simulink model "QPSK_delayChannel"  (R2017b)
settings: Solver=FixedStepDiscrete  StartTime=0.0  StopTime=inf  RelTol=1e-3
PreLoadFcn:
  | sdrqpsktx = sdrzqpsktxFMC234_init;
  | sdrqpskrx = sdrzqpskrxFMC234_init;
InitFcn:
  | sdrqpsktx = sdrzqpsktxFMC234_init;
  | sdrqpskrx = sdrzqpskrxFMC234_init;
undefined symbols (not defined in the file or in its folder): dfilt, gcbh, rcfiltgaincompat
libraries: commdigbbndpm3 x3, dspstat3 x3, dspobslib x3, dspsigops x2, commsequence2 x2, commutil2 x2, commfilt2 x2, simulink x2, commrfcorlib x1, commrflib2 x1, commblksprivate x1, dspspect3 x1
Description:
  | Implement a QPSK Transmitter prototype using SDR hardware
settings Model: FPTRunName=Active  ModifiedByFormat=The MathWorks Inc.  SimulationMode=accelerator  Creator=The MathWorks, Inc.  LastModifiedBy=The MathWorks Inc.
settings DataIOCC: LimitDataPoints=on  SaveFormat=Array  SaveOutput=off  SaveTime=off
settings OptimizationCC: BooleanDataType=off  DefaultParameterBehavior=Inlined  ExpressionDepthLimit=2147483647  LocalBlockOutputs=off  LifeSpan=inf
settings DebuggingCC: AlgebraicLoopMsg=error  UnderspecifiedInitializationDetection=Classic  MergeDetectMultiDrivingBlocksExec=none  SolverPrmCheckMsg=warning  SingleTaskRateTransMsg=error  FcnCallInpInsideContextMsg=warning  AllowSymbolicDim=off  StateNameClashWarn=warning  SFUnexpectedBacktrackingDiag=warning  SFNoUnconditionalDefaultTransitionDiag=warning  SFExecutionAtInitializationDiag=none
settings HardwareCC: ProdBitPerPointer=32  ProdBitPerSizeT=32  ProdBitPerPtrDiffT=32  ProdLargestAtomicFloat=None  ProdIntDivRoundTo=Undefined  ProdEndianess=Unspecified  ProdWordSize=32  ProdHWDeviceType=32-bit Generic  TargetBitPerPointer=64  TargetBitPerSizeT=64  TargetBitPerPtrDiffT=64  TargetLongLongMode=on  TargetIntDivRoundTo=Zero  TargetEndianess=LittleEndian  TargetWordSize=64  TargetHWDeviceType=Generic->MATLAB Host Computer  ProdEqTarget=off
settings ModelReferenceCC: PropagateSignalLabelsOutOfModel=off
settings RTWCC: CustomSourceCode=|
  | #include <stdio.h>
  | #include <stdlib.h>
settings CodeAppCC: StateflowObjectComments=on
settings GRTTargetCC: TargetLangStandard=C89/C90 (ANSI)  GeneratePreprocessorConditionals=Disable all  CombineOutputUpdateFcns=off  GRTInterface=on
settings ConfigComp: CovMetricSettings=dw  CovHtmlReporting=on  CovSaveCumulativeToWorkspaceVar=on  CovSaveSingleToWorkspaceVar=on  CovExternalEMLEnable=off  CovSFcnEnable=off

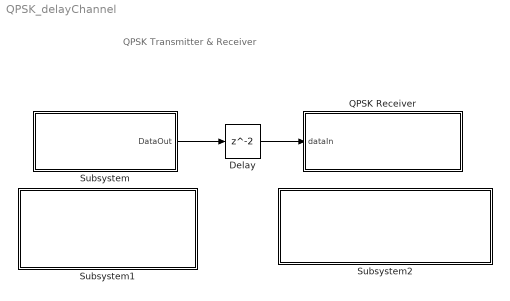
== system QPSK_delayChannel ==
  note: QPSK Transmitter & Receiver
  Delay : Delay  InitialCondition=0
  QPSK Receiver : Subsystem
      mask Display: disp('QPSK Receiver')
  Subsystem : Subsystem
      mask Display: disp('QPSK Transmitter')
  Subsystem1 : Subsystem
      mask init:
      | txStat = sdrzqpsktxFMC234_init;
      | rxStat = sdrzqpskrxFMC234_init;
      mask Display:
      | disp(['Sampling Frequency = ',num2str(txStat.Fs*1e-6),' MHz\n\n\n\n'])
      | disp(['Frame size = ',num2str(txStat.FrameSize),'\n\n'])
      | disp(['\n\nUpsampling Factor = ',num2str(txStat.Upsampling),'\n\n'])
      | disp('\n\n\n\n\n Transmitter Specifications')
  Subsystem2 : Subsystem
      mask init:
      | txStat = sdrzqpsktxFMC234_init;
      | rxStat = sdrzqpskrxFMC234_init;
      mask Display:
      | disp(['Sampling Frequency = ',num2str(rxStat.Fs*1e-6),' MHz\n\n'])
      | disp(['Radio Center Frequency = ',num2str(rxStat.RadioCenterFrequency*1e-9),' GHz\n\n\n\n'])
      | disp(['Frame size = ',num2str(rxStat.FrameSize)])
      | disp(['\n\nDownsampling & UpSampling Factor = ',num2str(rxStat.Downsampling), ' & ', num2str(rxStat.Upsampling)])
      | disp('\n\n\n\n\n Receiver Specifications')
  wires:
  Subsystem/1(DataOut) -> Delay/1
  Delay/1 -> QPSK Receiver/1(dataIn)

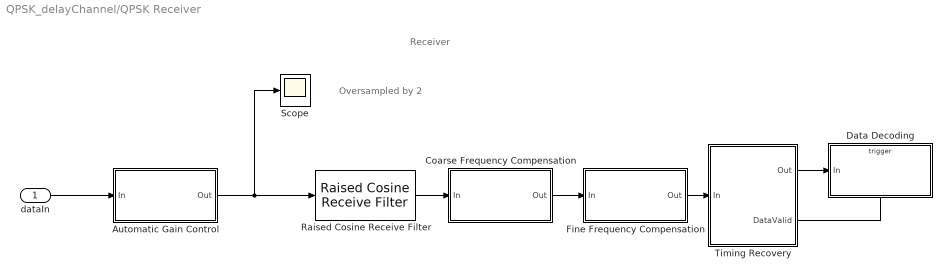
== system QPSK_delayChannel/QPSK Receiver ==
  note: Oversampled by 2
  note: Receiver
  dataIn : Inport
  Automatic Gain Control : Subsystem  mask{DesiredAmplitude=1/sqrt(sdrqpskrx.Upsampling)}
      mask prompts: DesiredAmplitude "Desired Amplitude"
      mask Display: disp('Automatic Gain\nControl')
  Coarse Frequency Compensation : Subsystem
      mask Display: disp('Coarse Frequency\nCompensation');
  Data Decoding : Subsystem
      mask Display: disp('Data Decoding');
  Fine Frequency Compensation : Subsystem
      mask Display: disp('Fine Frequency\nCompensation')
  Raised Cosine Receive Filter : commfilt2/Raised Cosine Receive Filter  filtType=Square root  R=0.5  filtSpan=sdrqpskrx.RCFiltSpan  N=sdrqpskrx.Upsampling  downFactor=sdrqpskrx.Downsampling  downOffset=0  filterGain=1  RateOptions=Allow multirate processing  framing=Mute  checkCoeff=off  variableName=rcRxFilt1  currentFiltSpan=sdrqpskrx.RCFiltSpan  D=(sdrqpskrx.RCFiltSpan)/2  inputOffset=0  sampMode=Mute  saveAsFlag=0  rateMode=Downsampling  checkGain=Normalized  launchFVT=off  roundingMode=Floor  overflowMode=off  coeffDataTypeStr=Inherit: Same word length as input  coeffMin=[]  coeffMax=[]  coeffLastDataTypeStr=Inherit: Same word length as input  accumDataTypeStr=Inherit: Same as product output  accumLastDataTypeStr=Inherit: Same as product output  outputDataTypeStr=Inherit: Same as accumulator  outputMin=[]  outputMax=[]  outputLastDataTypeStr=Inherit: Same as accumulator
  Scope : Scope
  Timing Recovery : Subsystem
      mask Display:
      | disp('Timing\nRecovery');
      | port_label('output',1,'DataOut');
      | port_label('output',2,'DataValid');
  wires:
  Timing Recovery/1(Out) -> Data Decoding/1(In)
  Timing Recovery/2(DataValid) -> Data Decoding/Trigger
  Raised Cosine Receive Filter/1 -> Coarse Frequency Compensation/1(In)
  Coarse Frequency Compensation/1(Out) -> Fine Frequency Compensation/1(In)
  Fine Frequency Compensation/1(Out) -> Timing Recovery/1(In)
  Automatic Gain Control/1(Out) -> Scope/1, Raised Cosine Receive Filter/1
  dataIn/1 -> Automatic Gain Control/1(In)

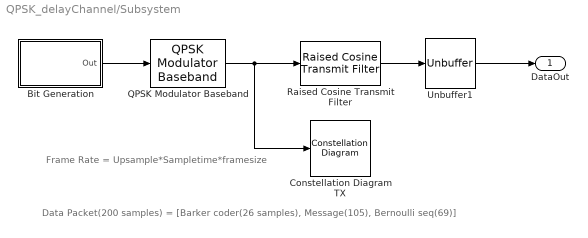
== system QPSK_delayChannel/Subsystem ==
  note: Data Packet(200 samples) = [Barker coder(26 samples), Message(105), Bernoulli seq(69)]
  note: Frame Rate = Upsample*Sampletime*framesize
  Bit Generation : Subsystem
      mask Display: disp('Bits Generation')
  Constellation Diagram TX : ConstellationDiagram
  QPSK Modulator Baseband : commdigbbndpm3/QPSK Modulator Baseband  InType=Bit  Enc=Gray  Ph=pi/4  outDtype=double  outWordLen=16  outUDDataType=sfix(16)  outFracLenMode=Best precision  outFracLen=15  outDataTypeStr=double  outLastDataTypeStr=double
  Raised Cosine Transmit Filter : commfilt2/Raised Cosine Transmit Filter  filtType=Square root  R=0.5  filtSpan=2*((sdrqpsktx.RCFiltSpan)/2)  N=sdrqpsktx.Upsampling  filterGain=rcfiltgaincompat(gcbh)  InputProcessing=Columns as channels (frame based)  RateOptions=Enforce single-rate processing  framing=Mute  checkCoeff=off  variableName=rcTxFilt1  checkGain=Normalized  sampMode=Mute  saveAsFlag=0  currentFiltSpan=2*((sdrqpsktx.RCFiltSpan)/2)  D=(sdrqpsktx.RCFiltSpan)/2  launchFVT=off  roundingMode=Floor  overflowMode=off  coeffDataTypeStr=Inherit: Same word length as input  coeffMin=[]  coeffMax=[]  coeffLastDataTypeStr=Inherit: Same word length as input  outputDataTypeStr=Inherit: Same as accumulator  outputMin=[]  outputMax=[]  outputLastDataTypeStr=Inherit: Same as accumulator
  Unbuffer1 : Unbuffer
  DataOut : Outport
  wires:
  Raised Cosine Transmit Filter/1 -> Unbuffer1/1
  QPSK Modulator Baseband/1 -> Constellation Diagram TX/1, Raised Cosine Transmit Filter/1
  Unbuffer1/1 -> DataOut/1
  Bit Generation/1(Out) -> QPSK Modulator Baseband/1

== system QPSK_delayChannel/Subsystem1 ==

== system QPSK_delayChannel/Subsystem2 ==

== system QPSK_delayChannel/QPSK Receiver/Automatic Gain Control ==
  In : Inport
  AGC : commrfcorlib/AGC  LegacyMode=off  DetectorMethod=Rectifier  LoopMethod=Linear  UpdatePeriod=40  StepSize=0.1  AdaptationStepSize=(0.1)/(40)  DesiredOutputPower=1  AveragingLength=40  MaximumGain=1e6  MaxPowerGain=2*(1e6)  GainOutputPort=off  InputPowerOutputPort=off  SimulateUsing=Interpreted execution
      settings: SourceProductName=Communications System Toolbox
  Gain : Gain  Gain=DesiredAmplitude
  Out : Outport
  wires:
  In/1 -> AGC/1
  AGC/1 -> Gain/1
  Gain/1 -> Out/1

== system QPSK_delayChannel/QPSK Receiver/Coarse Frequency Compensation ==
  In : Inport
  Compensate for Frequency Offset : commrflib2/Phase// Frequency Offset  phaseOffset=0  freqPort=on  freqOffset=100
      settings: SourceProductName=Communications System Toolbox
  Find Frequency Offset : Subsystem  mask(Find Frequency Offset){M=sdrqpskrx.M, fftLen=2048, fftAvgs=16}
      mask prompts: M "Modulation order (integer):"; fftLen "FFT length (integer):"; fftAvgs "FFT averages (integer):"
  Out : Outport
  wires:
  In/1 -> Compensate for Frequency Offset/1, Find Frequency Offset/1(In)
  Compensate for Frequency Offset/1 -> Out/1
  Find Frequency Offset/1(Frq) -> Compensate for Frequency Offset/2

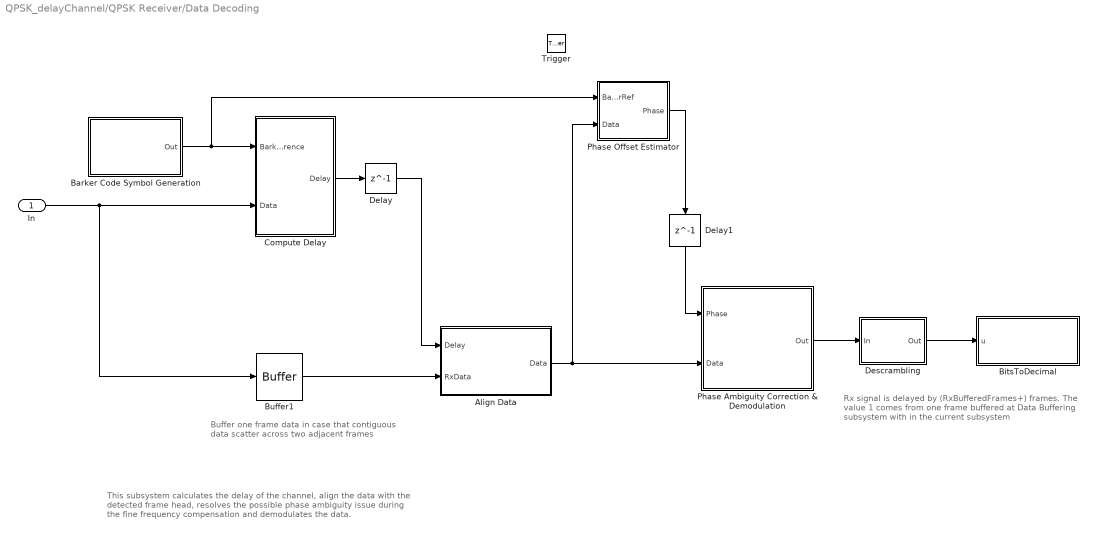
== system QPSK_delayChannel/QPSK Receiver/Data Decoding ==
  note: Buffer one frame data in case that contiguous
      | data scatter across two adjacent frames
  note: This subsystem calculates the delay of the channel, align the data with
      | the detected frame head, resolves the possible phase ambiguity issue
      | during the fine frequency compensation and demodulates the data.
  note: Rx signal is delayed by (RxBufferedFrames+) frames.
      | The value 1 comes from one frame buffered at Data
      | Buffering subsystem with in the current subsystem
  In : Inport
  Trigger : TriggerPort  VariantControl=Variant  PortDimensions=1
  Align Data : MATLAB Function  TreatAsAtomicUnit=on
  "Barker Code Symbol Generation " : Subsystem
      mask Display: disp('Barker Code\nSymbol Generation')
  BitsToDecimal : MATLAB Function  TreatAsAtomicUnit=on
  Buffer1 : Buffer  N=sdrqpskrx.FrameSize*2  V=sdrqpskrx.FrameSize  OutputFrames=off
  Compute Delay : Subsystem
      mask Display: disp('Compute\nDelay');
  Delay : Delay  DelayLength=1
  Delay1 : Delay  DelayLength=1
  Descrambling : Subsystem
      mask Display: disp('Descrambling')
  Phase Ambiguity Correction & Demodulation : Subsystem
      mask Display: disp('Phase Ambiguity\nCorrection\n& Demodulation');
  Phase Offset Estimator : Subsystem
  wires:
  Delay/1 -> Align Data/1(Delay)
  Buffer1/1 -> Align Data/2(RxData)
  In/1 -> Buffer1/1, Compute Delay/2(Data)
  Compute Delay/1(Delay) -> Delay/1
  Align Data/1(Data) -> Phase Ambiguity Correction & Demodulation/2(Data), Phase Offset Estimator/2(Data)
  Phase Ambiguity Correction & Demodulation/1(Out) -> Descrambling/1(In)
  "Barker Code Symbol Generation "/1(Out) -> Compute Delay/1(Barker Reference), Phase Offset Estimator/1(BarkerRef)
  Phase Offset Estimator/1(Phase) -> Delay1/1
  Delay1/1 -> Phase Ambiguity Correction & Demodulation/1(Phase)
  Descrambling/1(Out) -> BitsToDecimal/1(u)

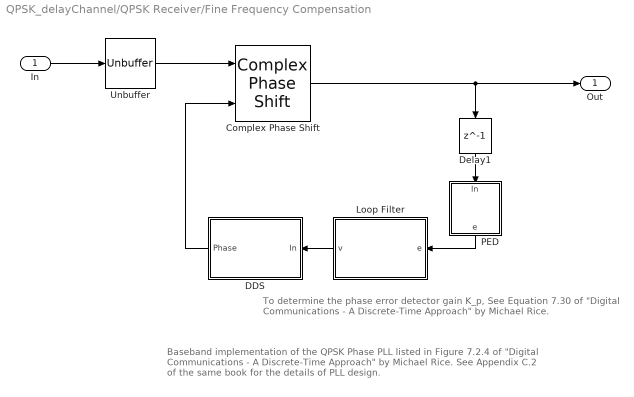
== system QPSK_delayChannel/QPSK Receiver/Fine Frequency Compensation ==
  note: To determine the phase error detector gain K_p, See Equation 7.30 of "Digital
      | Communications - A Discrete-Time Approach" by Michael Rice.
  note: Baseband implementation of the QPSK Phase PLL listed in Figure 7.2.4 of
      | "Digital Communications - A Discrete-Time Approach" by Michael Rice. See
      | Appendix C.2 of the same book for the details of PLL design.
  In : Inport
  Complex Phase Shift : commutil2/Complex Phase Shift
      settings: SourceProductName=Communications System Toolbox  SourceProductBaseCode=CM
  DDS : Subsystem
      mask Display: disp('DDS')
  Delay1 : Delay  DelayLength=1  InitialCondition=0  InputProcessing=Columns as channels (frame based)
  Loop Filter : Subsystem  mask{BnTs=0.06, zeta=2.5, N=sdrqpskrx.Upsampling/sdrqpskrx.Downsampling, Kp=sdrqpskrx.FineFreqPEDGain, K0=sdrqpskrx.FineFreqCompensateGain}
      mask prompts: BnTs "Normalized Loop Bandwidth"; zeta "Damping Factor"; N "Number of Samples/Symbol"; Kp "Phase Detector Gain (Kp)"; K0 "DDS Gain (K0)"
      mask init:
      | % See C.57 to C.61 in Michael Rice's "Digital Communications 
      | % - A Discrete-Time Approach" for details
      | theta = BnTs/(zeta+0.25/zeta)/N;
      | d = 1 + 2*zeta*theta + theta*theta;
      | K1 = 4*zeta*theta/d;
      | K2 = 4*theta*theta/d;
      | K1 = K1/(Kp*K0);
      | K2 = K2/(Kp*K0);
      mask Display: disp('Loop Filter')
  PED : MATLAB Function  TreatAsAtomicUnit=on
  Unbuffer : Unbuffer
  Out : Outport
  wires:
  PED/1(e) -> Loop Filter/1(e)
  Loop Filter/1(v) -> DDS/1(In)
  DDS/1(Phase) -> Complex Phase Shift/2
  Unbuffer/1 -> Complex Phase Shift/1
  In/1 -> Unbuffer/1
  Complex Phase Shift/1 -> Delay1/1, Out/1
  Delay1/1 -> PED/1(In)

== system QPSK_delayChannel/QPSK Receiver/Timing Recovery ==
  note: Baseband implementation of the Symbol Timing Synchronization listed in Chapter 8.4
      | of "Digital Communications- A Discrete-Time Approach" by Michael Rice. See
      | Appendix C.2 of the same book for the details of PLL design.
  note: MATLAB Implementation
      | of Scalar-based Timing Recovery
  In : Inport
  Modified Buffer : Subsystem  TreatAsAtomicUnit=on  mask(Input-Driven Buffer){bufSize=sdrqpskrx.FrameSize}
      mask prompts: bufSize "Buffer size:"
      mask help: A modified buffer subsystem that is driven by the arrival of its input data; it produces a valid output data buffer whenever its buffer is full and sets its dataValid flag to 1. Otherwise, the data at its dataOut port is not valid and its dataValid flag is set to 0.
  Timing Recovery PLL : Subsystem
      mask Display:
      | disp('Timing Recovery\nPLL')
      | port_label('input',1,'In')
      | port_label('output',1,'DataOut')
      | port_label('output',2,'Clk')
  Out : Outport
  DataValid : Outport  Port=2
  wires:
  Timing Recovery PLL/2(ClkOut) -> Modified Buffer/2(Clk)
  Timing Recovery PLL/1(DataOut) -> Modified Buffer/1(Data)
  In/1 -> Timing Recovery PLL/1(DataIn)
  Modified Buffer/1(DataOut) -> Out/1
  Modified Buffer/2(DataValid) -> DataValid/1

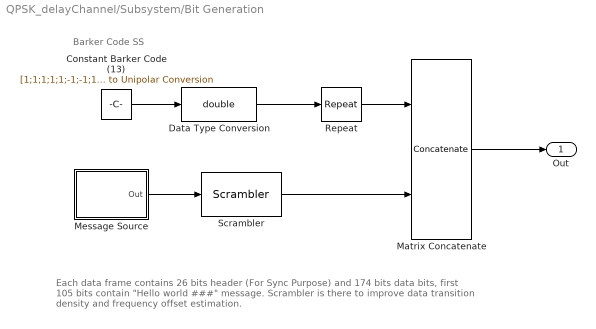
== system QPSK_delayChannel/Subsystem/Bit Generation ==
  note: Barker Code SS
  note: Each data frame contains 26 bits header (For Sync Purpose) and 174 bits data bits,
      | first 105 bits contain "Hello world ###" message. Scrambler is there to improve data
      | transition density and frequency offset estimation.
  Constant Barker Code (13) : Constant  Value=|
      | [1;1;1;1;1;-1;-1;1;1;-1;1;-1;1
      | ] > 0  % Bipolar to Unipolar Conversion
  Data Type Conversion : DataTypeConversion  OutDataTypeStr=double
  Matrix Concatenate : Concatenate  Mode=Multidimensional array
  Message Source : Subsystem
      mask Display: disp('Message\nSource')
  Repeat : dspsigops/Repeat  N=2  InputProcessing=Columns as channels (frame based)  RateOptions=Enforce single-rate processing  ic=0  mode=Unused parameter value
      settings: SourceProductName=DSP System Toolbox
  Scrambler : commsequence2/Scrambler  M=2  poly=[1 1 1 0 1]  iniStaSource=Dialog Parameter  ini_sta=[0 0 0 0]  resetViaPort=off
      settings: SourceProductName=Communications System Toolbox  SourceProductBaseCode=CM
  Out : Outport
  wires:
  Matrix Concatenate/1 -> Out/1
  Message Source/1(Out) -> Scrambler/1
  Repeat/1 -> Matrix Concatenate/1
  Scrambler/1 -> Matrix Concatenate/2
  Data Type Conversion/1 -> Repeat/1
  Constant Barker Code (13)/1 -> Data Type Conversion/1

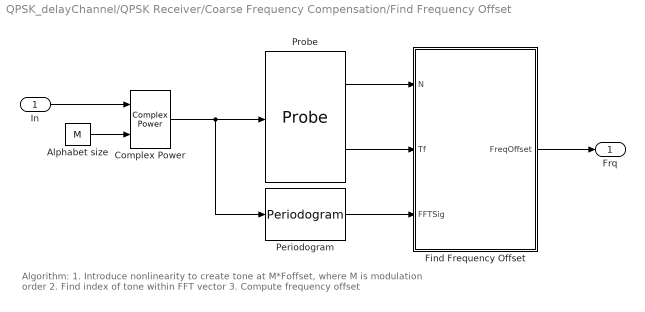
== system QPSK_delayChannel/QPSK Receiver/Coarse Frequency Compensation/Find Frequency Offset ==
  note: Algorithm:
      | 1.  Introduce nonlinearity to create tone at M*Foffset, where M is modulation order
      | 2.  Find index of tone within FFT vector
      | 3.  Compute frequency offset
  In : Inport
  Alphabet size : Constant  Value=M  OutDataTypeStr=Inherit: Inherit via back propagation
  Complex Power : commblksprivate/Complex Power
      settings: SourceProductName=Communications System Toolbox  SourceProductBaseCode=CM
  Find Frequency Offset : MATLAB Function  TreatAsAtomicUnit=on
  Periodogram : dspspect3/Periodogram  measurement=Power spectral density  wintype=Hamming  Rs=50  beta=5  winsamp=Symmetric  FFTImplementation=Auto  inheritFFT=off  fftsize=2048  navg=16  inheritTs=on  Ts=1
      settings: SourceProductName=DSP System Toolbox  SourceProductBaseCode=DS
  Probe : Probe  ProbeComplexSignal=off
  Frq : Outport
  wires:
  Periodogram/1 -> Find Frequency Offset/3(FFTSig)
  Alphabet size/1 -> Complex Power/2
  In/1 -> Complex Power/1
  Probe/1 -> Find Frequency Offset/1(N)
  Probe/2 -> Find Frequency Offset/2(Tf)
  Find Frequency Offset/1(FreqOffset) -> Frq/1
  Complex Power/1 -> Probe/1, Periodogram/1

== system QPSK_delayChannel/QPSK Receiver/Data Decoding/Barker Code Symbol Generation  ==
  note: Regenerate a QPSK-modulated unipolar Barker code sequence
      | to be compared with the received data
  Constant Barker Code (13) : Constant  Value=|
      | [1;1;1;1;1;-1;-1;1;1;-1;1;-1;1
      | ] > 0  % Bipolar to Unipolar Conversion
  Data Type Conversion : DataTypeConversion  OutDataTypeStr=double
  QPSK Modulator Baseband : commdigbbndpm3/QPSK Modulator Baseband  InType=Bit  Enc=Gray  Ph=pi/4  outDtype=double  outWordLen=16  outUDDataType=sfix(16)  outFracLenMode=Best precision  outFracLen=15  outDataTypeStr=double  outLastDataTypeStr=double
  Repeat : dspsigops/Repeat  N=2  InputProcessing=Columns as channels (frame based)  RateOptions=Enforce single-rate processing  ic=0  mode=Unused parameter value
      settings: SourceProductName=DSP System Toolbox
  Out : Outport
  wires:
  Repeat/1 -> QPSK Modulator Baseband/1
  QPSK Modulator Baseband/1 -> Out/1
  Data Type Conversion/1 -> Repeat/1
  Constant Barker Code (13)/1 -> Data Type Conversion/1

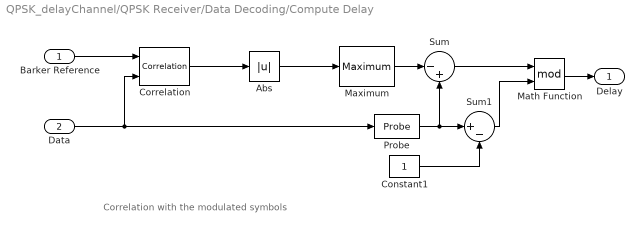
== system QPSK_delayChannel/QPSK Receiver/Data Decoding/Compute Delay ==
  note: Correlation with the modulated symbols
  Barker Reference : Inport
  Data : Inport  Port=2
  Abs : Abs
  Constant1 : Constant  VectorParams1D=off  OutDataTypeStr=Inherit: Inherit via back propagation  FramePeriod=2
  Correlation : dspstat3/Correlation  domain=Time  roundingMode=Floor  overflowMode=off  accumDataTypeStr=Inherit: Same as product output  accumLastDataTypeStr=Inherit: Same as product output  outputDataTypeStr=Inherit: Same as accumulator  outputMin=[]  outputMax=[]  outputLastDataTypeStr=Inherit: Same as accumulator
      settings: SourceProductName=DSP System Toolbox  SourceProductBaseCode=DS
  Math Function : Math  Operator=mod  SaturateOnIntegerOverflow=on
  Maximum : dspstat3/Maximum  operation=maximum  fcn=Index  indexBase=One  operateOver=Each column  Dimension=1  InputProcessing=Columns as channels (frame based)  reset=None  roiEnable=off  roiType=Rectangles  roiPortion=Entire ROI  roiOutput=Individual statistics for each ROI  roiFlag=off  roundingMode=Floor  overflowMode=off  accumDataTypeStr=Inherit: Same as product output  accumLastDataTypeStr=Inherit: Same as product output
  Probe : Probe  ProbeSampleTime=off  ProbeComplexSignal=off
  Sum : Sum  Inputs=|-+  SaturateOnIntegerOverflow=on  InputSameDT=on  OutDataTypeStr=Inherit: Same as first input
  Sum1 : Sum  Inputs=|+-  SaturateOnIntegerOverflow=on  InputSameDT=on  OutDataTypeStr=Inherit: Same as first input
  Delay : Outport
  wires:
  Abs/1 -> Maximum/1
  Constant1/1 -> Sum1/2
  Sum1/1 -> Math Function/2
  Math Function/1 -> Delay/1
  Sum/1 -> Math Function/1
  Probe/1 -> Sum1/1, Sum/2
  Correlation/1 -> Abs/1
  Maximum/1 -> Sum/1
  Barker Reference/1 -> Correlation/1
  Data/1 -> Correlation/2, Probe/1

== system QPSK_delayChannel/QPSK Receiver/Data Decoding/Descrambling ==
  In : Inport
  Descrambler : commsequence2/Descrambler  M=2  poly=[1 1 1 0 1]  iniStaSource=Dialog Parameter  ini_sta=[0 0 0 0]  resetViaPort=off
      settings: SourceProductName=Communications System Toolbox  SourceProductBaseCode=CM
  Selector : Selector  IndexOptions=Index vector (dialog)  Indices=[sdrqpskrx.BarkerLength*log2(sdrqpskrx.M)+1:sdrqpskrx.FrameSize*log2(sdrqpskrx.M)]  OutputSizes=1
  Selector1 : Selector  IndexOptions=Index vector (dialog)  Indices=[1:sdrqpskrx.MsgLength]  OutputSizes=1
  Out : Outport
  wires:
  Descrambler/1 -> Selector1/1
  Selector1/1 -> Out/1
  In/1 -> Selector/1
  Selector/1 -> Descrambler/1

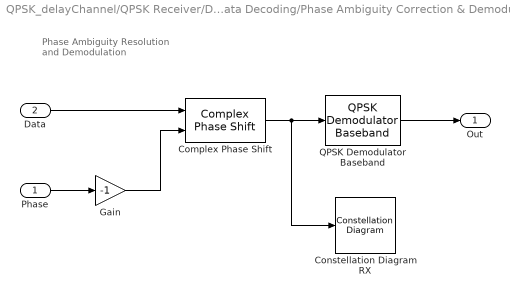
== system QPSK_delayChannel/QPSK Receiver/Data Decoding/Phase Ambiguity Correction & Demodulation ==
  note: Phase Ambiguity Resolution
      | and Demodulation
  Phase : Inport
  Data : Inport  Port=2
  Complex Phase Shift : commutil2/Complex Phase Shift
      settings: SourceProductName=Communications System Toolbox  SourceProductBaseCode=CM
  Constellation Diagram RX : ConstellationDiagram
  Gain : Gain  Gain=-1
  QPSK Demodulator Baseband : commdigbbndpm3/QPSK Demodulator Baseband  OutType=Bit  DecType=Hard decision  VarSource=Dialog  Variance=1  Dec=Gray  Ph=pi/4  outDtype1=Inherit via internal rule  outDtype2=Inherit via internal rule  derotateFactorWordLen=16  derotateFactorDataTypeStr=Inherit: Same word length as input  derotateFactorLastDataTypeStr=Inherit: Same word length as input
  Out : Outport
  wires:
  Phase/1 -> Gain/1
  Data/1 -> Complex Phase Shift/1
  Complex Phase Shift/1 -> Constellation Diagram RX/1, QPSK Demodulator Baseband/1
  QPSK Demodulator Baseband/1 -> Out/1
  Gain/1 -> Complex Phase Shift/2

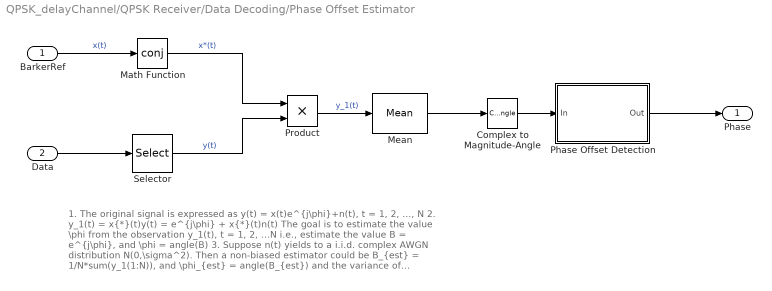
== system QPSK_delayChannel/QPSK Receiver/Data Decoding/Phase Offset Estimator ==
  note: 1. The original signal is expressed as y(t) = x(t)e^{j\phi}+n(t), t = 1, 2, ..., N
      | 2. y_1(t) = x{*}(t)y(t) = e^{j\phi} + x{*}(t)n(t)
      | The goal is to estimate the value \phi from the observation y_1(t), t = 1, 2, ...N
      | i.e., estimate the value B = e^{j\phi}, and \phi = angle(B)
      | 3. Suppose n(t) yields to a i.i.d. complex AWGN distribution N(0,\sigma^2).
      | Then a non-biased estimator could be
      | B_{est} = 1/N*sum(y_1(1:N)), and \phi_{est} = angle(B_{est})
      | and the variance of B_{est} is \sigma^2/N
  BarkerRef : Inport
  Data : Inport  Port=2
  Complex to Magnitude-Angle : ComplexToMagnitudeAngle  Output=Angle
  Math Function : Math  Operator=conj  SaturateOnIntegerOverflow=on
  Mean : dspstat3/Mean  run=off  reset_popup=None  InputProcessing=Columns as channels (frame based)  directionMode=Each column  dimension=1  roiEnable=off  roiType=Rectangles  roiPortion=Entire ROI  roiOutput=Individual statistics for each ROI  roiFlag=off  outputDataTypeStr=Inherit: Same as accumulator  outputLastDataTypeStr=Inherit: Same as accumulator  outputMin=[]  outputMax=[]  roundingMode=Floor  overflowMode=off
  Phase Offset Detection : MATLAB Function  TreatAsAtomicUnit=on
  Product : Product  RndMeth=Zero
  Selector : Selector  IndexOptions=Index vector (dialog)  Indices=[1:sdrqpskrx.BarkerLength]  OutputSizes=1
  Phase : Outport
  wires:
  Data/1 -> Selector/1
  BarkerRef/1 -> Math Function/1  "x(t)"
  Selector/1 -> Product/2  "y(t)"
  Math Function/1 -> Product/1  "x*(t)"
  Product/1 -> Mean/1  "y_1(t)"
  Mean/1 -> Complex to Magnitude-Angle/1
  Complex to Magnitude-Angle/1 -> Phase Offset Detection/1(In)
  Phase Offset Detection/1(Out) -> Phase/1

== system QPSK_delayChannel/QPSK Receiver/Fine Frequency Compensation/DDS ==
  note: The digital filter acts as a pure integrator
  In : Inport
  Digital Filter : dspobslib/Digital Filter  TypePopup=IIR (poles & zeros)  IIRFiltStruct=Direct form II transposed  AllPoleFiltStruct=Direct form  FIRFiltStruct=Direct form  CoeffSource=Specify via dialog  NumCoeffs=[0 1]  DenCoeffs=[1 -1]  BiQuadCoeffs=[1 0.3 0.4 1 0.1 0.2]  LatticeCoeffs=[0.2 0.4]  denIgnore=on  FiltPerSampPopup=One filter per frame  IC=0  ICnum=0  ICden=0  roundingMode=Floor  overflowMode=off  ScaleValues=1  scaleValueFracLength=14  stageInFracLength=15  stageOutFracLength=15  FilterSource=Specify via dialog  dfiltObjectName=dfilt.dffir([1 2 1])  InputProcessing=Columns as channels (frame based)
      settings: SourceProductName=DSP System Toolbox  SourceProductBaseCode=DS
  Gain : Gain  Gain=-1*sdrqpskrx.FineFreqCompensateGain
  Phase : Outport
  wires:
  Digital Filter/1 -> Gain/1
  In/1 -> Digital Filter/1
  Gain/1 -> Phase/1

== system QPSK_delayChannel/QPSK Receiver/Fine Frequency Compensation/Loop Filter ==
  note: Proportional-plus-Integrator Loop Filter,
      | Infinite DC Response to guarantee convergence
  e : Inport
  Digital Filter : dspobslib/Digital Filter  TypePopup=IIR (poles & zeros)  IIRFiltStruct=Direct form II transposed  AllPoleFiltStruct=Direct form  FIRFiltStruct=Direct form  CoeffSource=Specify via dialog  NumCoeffs=[1 0]  DenCoeffs=[1 -1]  BiQuadCoeffs=[1 0.3 0.4 1 0.1 0.2]  LatticeCoeffs=[0.2 0.4]  denIgnore=on  FiltPerSampPopup=One filter per frame  IC=0  ICnum=0  ICden=0  roundingMode=Floor  overflowMode=off  ScaleValues=1  scaleValueFracLength=14  stageInFracLength=15  stageOutFracLength=15  FilterSource=Specify via dialog  dfiltObjectName=dfilt.dffir([1 2 1])  InputProcessing=Columns as channels (frame based)
      settings: SourceProductName=DSP System Toolbox  SourceProductBaseCode=DS
  K1 : Gain  Gain=K1
  K2 : Gain  Gain=K2
  Sum2 : Sum  SaturateOnIntegerOverflow=on  InputSameDT=on  OutDataTypeStr=Inherit: Same as first input
  v : Outport
  wires:
  K2/1 -> Digital Filter/1
  Digital Filter/1 -> Sum2/2
  Sum2/1 -> v/1
  e/1 -> K2/1, K1/1
  K1/1 -> Sum2/1

== system QPSK_delayChannel/QPSK Receiver/Timing Recovery/Modified Buffer ==
  Data : Inport
  Clk : Inport  Port=2
  Logical Operator : Logic  AllPortsSameDT=off  OutDataTypeStr=boolean
  Modified Buffer : Subsystem
  DataOut : Outport
  DataValid : Outport  Port=2
  wires:
  Data/1 -> Modified Buffer/1(In1)
  Clk/1 -> Modified Buffer/Enable, Logical Operator/2
  Modified Buffer/1(DataOut) -> DataOut/1
  Modified Buffer/2(DataValid) -> Logical Operator/1
  Logical Operator/1 -> DataValid/1

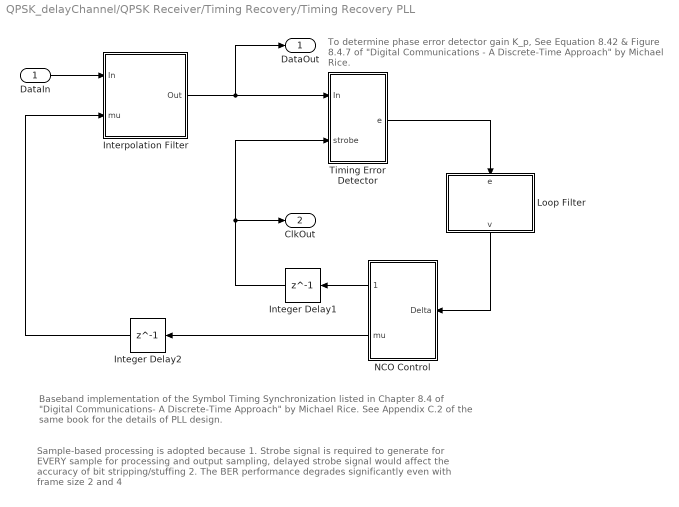
== system QPSK_delayChannel/QPSK Receiver/Timing Recovery/Timing Recovery PLL ==
  note: Sample-based processing is adopted because
      | 1. Strobe signal is required to generate for EVERY sample for processing and output
      | sampling, delayed strobe signal would affect the accuracy of bit stripping/stuffing
      | 2. The BER performance degrades significantly even with frame size 2 and 4
  note: Baseband implementation of the Symbol Timing Synchronization listed in Chapter 8.4
      | of "Digital Communications- A Discrete-Time Approach" by Michael Rice. See Appendix
      | C.2 of the same book for the details of PLL design.
  note: To determine phase error detector gain K_p, See Equation 8.42 &
      | Figure 8.4.7 of "Digital Communications - A Discrete-Time Approach"
      | by Michael Rice.
  DataIn : Inport
  Integer Delay1 : Delay  DelayLength=1  InputProcessing=Inherited
  Integer Delay2 : Delay  DelayLength=1  InputProcessing=Inherited
  Interpolation Filter : MATLAB Function  TreatAsAtomicUnit=on
  Loop Filter : Subsystem  mask{BnTs=0.01, zeta=1, Kp=sdrqpskrx.TimingRecTEDGain, K0=sdrqpskrx.TimingRecCompensateGain, N=sdrqpskrx.Upsampling/sdrqpskrx.Downsampling}
      mask prompts: BnTs "Loop Bandwidth"; zeta "Loop Damping Factor"; Kp "Phase Detector Gain (Kp)"; K0 "DDS gain (K0)"; N "Number of Samples/symbol (N)"
      mask init:
      | % See C.57 to C.61 in Michael Rice's "Digital Communications 
      | % - A Discrete-Time Approach" for details
      | theta = BnTs/(zeta+0.25/zeta)/N;
      | d = 1 + 2*zeta*theta + theta*theta;
      | K1 = 4*zeta*theta/d;
      | K2 = 4*theta*theta/d;
      | K1 = K1/(Kp*K0);
      | K2 = K2/(Kp*K0);
      mask Display: disp('Loop Filter');
  NCO Control : MATLAB Function
  Timing Error Detector : MATLAB Function  TreatAsAtomicUnit=on
  DataOut : Outport
  ClkOut : Outport  Port=2
  wires:
  DataIn/1 -> Interpolation Filter/1(In)
  NCO Control/2(mu) -> Integer Delay2/1
  Integer Delay1/1 -> ClkOut/1, Timing Error Detector/2(strobe)
  NCO Control/1(Underflow) -> Integer Delay1/1
  Interpolation Filter/1(Out) -> DataOut/1, Timing Error Detector/1(In)
  Loop Filter/1(v) -> NCO Control/1(Delta)
  Timing Error Detector/1(e) -> Loop Filter/1(e)
  Integer Delay2/1 -> Interpolation Filter/2(mu)

== system QPSK_delayChannel/Subsystem/Bit Generation/Message Source ==
  Bernoulli Binary Generator1 : commrandsrc3/Bernoulli Binary Generator  ProbabilityOfZero=0.5  SeedSource=Parameter  Seed=61  SampleTime=sdrqpsktx.FrameTime/(sdrqpsktx.DataLength-sdrqpsktx.MsgLength)  SamplesPerFrame=sdrqpsktx.DataLength-sdrqpsktx.MsgLength  OutputDataType=double  SimulateUsing=Interpreted execution
  Matrix Concatenate : Concatenate  Mode=Multidimensional array
  Message Generator : MATLAB Function  TreatAsAtomicUnit=on
  Out : Outport
  wires:
  Message Generator/1(msg) -> Matrix Concatenate/1
  Bernoulli Binary Generator1/1 -> Matrix Concatenate/2
  Matrix Concatenate/1 -> Out/1

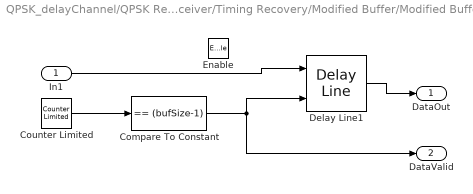
== system QPSK_delayChannel/QPSK Receiver/Timing Recovery/Modified Buffer/Modified Buffer ==
  In1 : Inport
  Enable : EnablePort
  Compare To Constant : simulink/Logic and Bit Operations/Compare To Constant  relop===  const=(bufSize-1)  OutDataTypeStr=boolean  ZeroCross=off
  Counter Limited : simulink/Sources/Counter Limited  uplimit=(bufSize-1)  tsamp=-1
  Delay Line1 : dspbuff3/Delay Line  siz=bufSize  ic=0  directfeed=on  enable_output=on  hold_output=off  OutputFrames=off
      settings: SourceProductName=DSP System Toolbox  SourceProductBaseCode=DS
  DataOut : Outport
  DataValid : Outport  Port=2
  wires:
  Compare To Constant/1 -> Delay Line1/2, DataValid/1
  Delay Line1/1 -> DataOut/1
  In1/1 -> Delay Line1/1
  Counter Limited/1 -> Compare To Constant/1

== system QPSK_delayChannel/QPSK Receiver/Timing Recovery/Timing Recovery PLL/Loop Filter ==
  note: Proportional-Plus-Integrator Loop Filter,
      | Infinite DC Response to guarantee convergence
  e : Inport
  Digital Filter : dspobslib/Digital Filter  TypePopup=IIR (poles & zeros)  IIRFiltStruct=Direct form II transposed  AllPoleFiltStruct=Direct form  FIRFiltStruct=Direct form  CoeffSource=Specify via dialog  NumCoeffs=[1 0]  DenCoeffs=[1 -1]  BiQuadCoeffs=[1 0.3 0.4 1 0.1 0.2]  LatticeCoeffs=[0.2 0.4]  denIgnore=on  FiltPerSampPopup=One filter per frame  IC=0  ICnum=0  ICden=0  roundingMode=Floor  overflowMode=off  ScaleValues=1  scaleValueFracLength=14  stageInFracLength=15  stageOutFracLength=15  FilterSource=Specify via dialog  dfiltObjectName=dfilt.dffir([1 2 1])  InputProcessing=Columns as channels (frame based)
      settings: SourceProductName=DSP System Toolbox  SourceProductBaseCode=DS
  K1 : Gain  Gain=K1
  K2 : Gain  Gain=K2
  Sum2 : Sum  SaturateOnIntegerOverflow=on  InputSameDT=on  OutDataTypeStr=Inherit: Same as first input
  v : Outport
  wires:
  K2/1 -> Digital Filter/1
  Digital Filter/1 -> Sum2/2
  Sum2/1 -> v/1
  e/1 -> K2/1, K1/1
  K1/1 -> Sum2/1

== matlab function QPSK_delayChannel/QPSK Receiver/Coarse Frequency Compensation/Find Frequency Offset/Find Frequency Offset ==
  data: N input; FreqOffset output; Tf input; FFTSig input; M parameter
 function FreqOffset = findfreqoffset(N,Tf,FFTSig,M) %#codegen
%  Estimate frequency offset.
%  findfreqoffset(N,Tf,fvec,params) returns the estimated frequency offset
%  given time-domain frame length N, sample time vector Tf containing
%  [frameTime,offsetTime], complex FFT vector FFTsig, and modulation
%  order M.

% Find index of max magnitude, convert to offset symmetric about zero.
% Return a negative integer offset to be interpreted as a compensation.
[~,maxIdx] = max(FFTSig);
FFTSize = size(FFTSig,1);
if maxIdx > FFTSize/2
    OffsetIdx = FFTSize+1-maxIdx;
else
    OffsetIdx = 1-maxIdx;
end
% Map offset index to a frequency value.
% Compute offset using modulation alphabet size params.M.
Ts = Tf(1)/N; % Sample time
delta_f = 1/(Ts*FFTSize); % Frequency resolution of FFT
FreqOffset = OffsetIdx * delta_f / M;

== matlab function QPSK_delayChannel/QPSK Receiver/Data Decoding/Align Data ==
  data: Delay input; Data output; RxData input
function Data  = aligndata(Delay, RxData)
% Extract data from the buffered RxData, using the delay to find the frame 
% start
%
% Input:
% Delay - Index of frame start
% RxData - Buffered symbol-spaced data
% Output:
% Data - Data with the Barker code at frame start
%#codegen
Data = RxData(Delay+1:Delay+length(RxData)/2);

== matlab function QPSK_delayChannel/Subsystem/Bit Generation/Message Source/Message Generator ==
  data: msg output
function msg = genMsg
%#codegen
persistent msgStrSet count;
if isempty(msgStrSet)
    count = 0;
    msgStrSet = ['Hello world 000';...
              'Hello world 001';...
              'Hello world 002';...
              'Hello world 003';...
              'Hello world 004';...
              'Hello world 005';...
              'Hello world 006';...
              'Hello world 007';...
              'Hello world 008';...
              'Hello world 009';...
              'Hello world 010';...
              'Hello world 011';...
              'Hello world 012';...
              'Hello world 013';...
              'Hello world 014';...
              'Hello world 015';...
              'Hello world 016';...
              'Hello world 017';...
              'Hello world 018';...
              'Hello world 019';...
              'Hello world 020';...
              'Hello world 021';...
              'Hello world 022';...
              'Hello world 023';...
              'Hello world 024';...
              'Hello world 025';...
              'Hello world 026';...
              'Hello world 027';...
              'Hello world 028';...
              'Hello world 029';...
              'Hello world 030';...
              'Hello world 031';...
              'Hello world 032';...
              'Hello world 033';...
              'Hello world 034';...
              'Hello world 035';...
              'Hello world 036';...
              'Hello world 037';...
              'Hello world 038';...
              'Hello world 039';...
              'Hello world 040';...
              'Hello world 041';...
              'Hello world 042';...
              'Hello world 043';...
              'Hello world 044';...
              'Hello world 045';...
              'Hello world 046';...
              'Hello world 047';...
              'Hello world 048';...
              'Hello world 049';...
              'Hello world 050';...
              'Hello world 051';...
              'Hello world 052';...
              'Hello world 053';...
              'Hello world 054';...
              'Hello world 055';...
              'Hello world 056';...
              'Hello world 057';...
              'Hello world 058';...
              'Hello world 059';...
              'Hello world 060';...
              'Hello world 061';...
              'Hello world 062';...
              'Hello world 063';...
              'Hello world 064';...
              'Hello world 065';...
              'Hello world 066';...
              'Hello world 067';...
              'Hello world 068';...
              'Hello world 069';...
              'Hello world 070';...
              'Hello world 071';...
              'Hello world 072';...
              'Hello world 073';...
              'Hello world 074';...
              'Hello world 075';...
              'Hello world 076';...
              'Hello world 077';...
              'Hello world 078';...
              'Hello world 079';...
              'Hello world 080';...
              'Hello world 081';...
              'Hello world 082';...
              'Hello world 083';...
              'Hello world 084';...
              'Hello world 085';...
              'Hello world 086';...
              'Hello world 087';...
              'Hello world 088';...
              'Hello world 089';...
              'Hello world 090';...
              'Hello world 091';...
              'Hello world 092';...
              'Hello world 093';...
              'Hello world 094';...
              'Hello world 095';...
              'Hello world 096';...
              'Hello world 097';...
              'Hello world 098';...
              'Hello world 099'];              
end
msgStr = msgStrSet(count+1,:);
msgBin = de2bi(int8(msgStr),7,'left-msb');
msg = reshape(double(msgBin).',105,1);
count = mod(count+1,100);

== matlab function QPSK_delayChannel/QPSK Receiver/Data Decoding/BitsToDecimal ==
  data: u input
function BitsToASCII(u)
% Convert bits to ASCII message.

coder.extrinsic('disp')

% Convert binary-valued column vector to 7-bit decimal values.
w = [64 32 16 8 4 2 1]; % binary digit weighting
Nbits = numel(u);
Ny = Nbits/7;
y = zeros(1,Ny);
for i = 0:Ny-1
    y(i+1) = w*u(7*i+(1:7));
end

% Display ASCII message to command window
disp(char(y));

== matlab function QPSK_delayChannel/QPSK Receiver/Data Decoding/Phase Offset Estimator/Phase Offset Detection ==
  data: In input; Out output
function Out = phasedecision(In)
% Map the estimated phase to one of -pi, -pi/2, 0, pi/2,  
%#codegen
% Out = round(In.*2./pi)./2.*pi;
% The above processing is equivalent to the following processing using
% if/else statements
%
% if In<pi/4 && In>-pi/4
%     Out = 0;
% elseif In>=pi/4 && In<pi*3/4
%     Out = pi/2;
% elseif In>=pi*3/4 || In<=-pi*3/4
%     Out = -pi;
% else
%     Out = -pi/2;
% end

if In<pi/4 && In>=-pi/4
    Out = 0;
elseif In>=pi/4 && In<pi*3/4
    Out = pi/2;
elseif In>=pi*3/4 || In<-pi*3/4
    Out = -pi;
else
    Out = -pi/2;
end

== matlab function QPSK_delayChannel/QPSK Receiver/Fine Frequency Compensation/PED ==
  data: In input; e output
function e = PED(In)
% Implementation of Maximum Likelihood Phase Error Detector listed in
% Chapter 7.2.2 of "Digital Communications - A Discrete-Time Approach" by
% Michael Rice. This employs a decision directed method.
% 
% Input: 
%   In - Input samples, oversampled by two
% Output:
%   e - Phase error, de
%#codegen

e = sign(real(In)).*imag(In) - sign(imag(In)).*real(In);

== matlab function QPSK_delayChannel/QPSK Receiver/Timing Recovery/Timing Recovery PLL/Interpolation Filter ==
  data: In input; Out output; mu input
function Out = interp_filter(In, mu)
% Prabolic piecewise polynomial interpolator, Farrow Interpolator with 
% alpha = 1/2, see Figure 8.4.16 of "Digital Communications - A 
% Discrete-Time Approach" by Michael Rice.
% Input:
%   In - Input samples, oversampled by two
%   mu - Difference between actual sampling instant and the optimal instant,
%        between zero and one
% Output:
%   Out - Interpolation output
%#codegen
persistent delay1 delay2 delay3; % Input delayed by 1, 2 and 3 samples
if isempty(delay1)
    [delay1, delay2, delay3] = deal(complex(0,0));
end

K = -0.5;

Out = delay2 + mu.*(K.*(In+delay2+delay3)+(1-K).*delay1)...
      + K.*(delay1+delay2-In-delay3).*mu.^2;
  
% Update delay buffers
delay3 = delay2;
delay2 = delay1;
delay1 = In;

== matlab function QPSK_delayChannel/QPSK Receiver/Timing Recovery/Timing Recovery PLL/NCO Control ==
  data: Delta input; Underflow output; mu output; sdrqpskrx parameter
function [Underflow, mu] = NCO_ctrl(Delta, sdrqpskrx)
% Implementation of modulo-1 counter for interpolation control listed in
% Figure 8.4.19 of "Digital Communications - A Discrete-Time Approach"
% by Michael Rice. See design details in Chapter 8.4.3 of the same book.
% 
% Input:
%   Delta - Loop filter output. If loop is in lock, delta would be small
%   qpsktxrx - Simulation parameter structure
% Output:
%   Underflow - Indicator of counter underflow. This is the strobe signal
%   for downstream processing
%   mu - Difference between actual sampling instant and the optimal instant,
%        between zero and one
%#codegen

% delay1 - Counter value delayed by 1 sample
% Regtemp - The estimated timing error normalized by half QPSK symbols
persistent delay1 Regtemp;  
if isempty(delay1)
    [delay1, Regtemp] = deal(0);
end
Upsampling = sdrqpskrx.Upsampling;
Downsampling = sdrqpskrx.Downsampling;
oversampling = Upsampling/Downsampling;

counter = mod(delay1,1)-Delta-1/oversampling; % decrementing counter
if counter < 0
    Underflow = 1;
    Regtemp = mod(delay1,1)/(Delta+1/oversampling);
else
    Underflow = 0;
end

mu = Regtemp;

% Update delay buffer
delay1 = mod(delay1,1)-Delta-1/oversampling;

== matlab function QPSK_delayChannel/QPSK Receiver/Timing Recovery/Timing Recovery PLL/Timing Error Detector ==
  data: In input; e output; strobe input
function e = TED(In, strobe)
% Zero-Crossing Timing Error Detector. See "Zero-Crossing Timing Error
% Detector" section in Chapter 8.4.1 of "Digital Communications - A
% Discrete-Time Approach" by Michael Rice. For bit stuffing/stripping
% details, see page 490-494 of the same book.
%
% Input: 
%   In - Input samples, interpolation result
%   strobe - Signal to enable timing error calculation
% Output:
%   e - Timing error
%#codegen
persistent delay1 delay2 delayStrobe; % Input delayed by one and 2 samples, and
% Enable signal delayed by one sample
if isempty(delay1)
    [delay1, delay2] = deal(complex(0,0));
    delayStrobe = 0;
end

if strobe==1 && delayStrobe~=strobe
    e = real(delay1) * (sign(real(delay2)) - sign(real(In))) + ...
        imag(delay1) * (sign(imag(delay2)) - sign(imag(In)));
else
    e = 0;
end

if delayStrobe~=strobe
    % Shift contents in delay register
    delay2 = delay1;
    delay1 = In;
elseif strobe==1
    % Two consecutive high strobes
    delay2 = 0; % Stuff missing sample
    delay1 = In; 
end
% If both current and previous enable signals are 0, skip current sample
% and keep the delayed signals unchanged. (Bit stripping)
delayStrobe = strobe;
